simulink model "KEYPAD_FIN"  (R2019b)
settings: Solver=ode1  StartTime=0.0  StopTime=150  FixedStep=0.001  RelTol=1e-3  EnableMultiTasking=on
undefined symbols (not defined in the file or in its folder): sigbuilder_block
settings Model: ExtModeTrigDuration=2  Creator=estra  LastModifiedBy=fabia
settings DataIOCC: ReturnWorkspaceOutputs=off
settings OptimizationCC: MaxStackSize=64  EfficientTunableParamExpr=on
settings DebuggingCC: ParameterTunabilityLossMsg=error  FrameProcessingCompatibilityMsg=warning  NonCurrentReleaseOperatingPointMsg=warning  ArithmeticOperatorsInVariantConditions=warning
settings HardwareCC: ProdBitPerInt=16  ProdBitPerPointer=16  ProdBitPerSizeT=16  ProdBitPerPtrDiffT=16  ProdLargestAtomicFloat=None  ProdWordSize=8  ProdHWDeviceType=Atmel->AVR
settings SFSimCC: SimUseLocalCustomCode=off  MATLABDynamicMemAlloc=off  CustomCodeUndefinedFunction=UseInterfaceOnly
settings RTWCC: SystemTargetFile=ert.tlc  HardwareBoard=Arduino Uno  TLCOptions=-aInlineSetEventsForThisBaseRateFcn=TLC_FALSE -aSuppressMultiTaskScheduler=TLC_FALSE -aRateBasedStepFcn=1  TemplateMakefile=ert_default_tmf  GenerateReport=on  RTWUseLocalCustomCode=off  Toolchain=Arduino AVR  BuildConfiguration=Faster Runs  IncludeHyperlinkInReport=on  LaunchReport=on  GenerateTraceInfo=on  GenerateTraceReport=on  GenerateTraceReportSl=on  GenerateTraceReportSf=on  GenerateTraceReportEml=on
settings CodeAppCC: ForceParamTrailComments=on  IgnoreCustomStorageClasses=off  OperatorAnnotations=on  SimulinkDataObjDesc=on  SFDataObjDesc=on  MATLABFcnDesc=on  InsertBlockDesc=on  StateflowObjectComments=on  MATLABSourceComments=on
settings ERTTargetCC: MultiwordLength=2048  SupportContinuousTime=on  SupportVariableSizeSignals=on

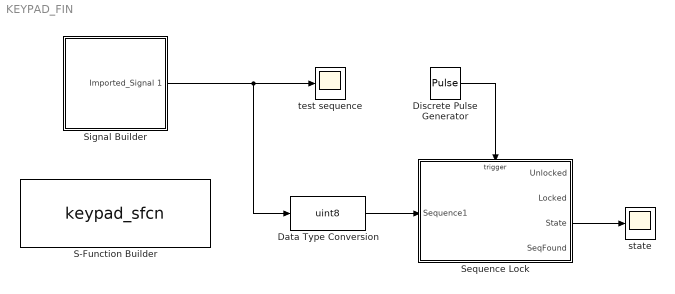
== system KEYPAD_FIN ==
  Data Type Conversion : DataTypeConversion  OutDataTypeStr=uint8
  Discrete Pulse Generator : DiscretePulseGenerator  PulseType=Time based  Period=0.01  PulseWidth=50
  S-Function Builder : S-Function  InitFcn=try, set_param(gcb,'FunctionName','keypad_sfcn'), end  FunctionName=keypad_sfcn  SFunctionModules=keypad_sfcn_wrapper  SFunctionDeploymentMode=off  EnableBusSupport=off  mask(S-Function Builder){}
      mask help: Simulink:masks:SFunctionBuilder_MD
      mask init:
      | val = [[.9  0.75 0.75 1 1 .9 .9 1]',[1 1 0.75 0.75 .9 .9 1 .9]'];try , sys = get_param(gcb,'SfunBuilderFcnName');if isempty(sys), sys = get_param(gcb,'FunctionName'); end,catch, sys = get_param(gcb,'FunctionName'); end
      settings: CopyFcn=set_param(gcbh,'LinkStatus','none')  PreSaveFcn=try, set_param(gcb,'FunctionName','keypad_sfcn'), end  OpenFcn=sfunctionwizard(gcbh)
      mask Display: plot(val(:,1),val(:,2)),disp(sys), port_label('output',1,'y0')
  Sequence Lock : Subsystem
  Signal Builder : Subsystem  Tag=STV Subsys  LoadFcn=sigbuilder_block('load');  StartFcn=sigbuilder_block('start');  StopFcn=sigbuilder_block('stop');  ClipboardFcn=sigbuilder_block('clipboard');  mask(Sigbuilder block){tuvar=[0:10]}
      mask help: Simulink:masks:SigbuilderBlock_MD
      mask init:
      | if ~strcmp(get_param(bdroot(gcbh),'SimulationStatus'),'stopped') tuvar = sigbuilder_block('maskInit'); end
      settings: CopyFcn=sigbuilder_block('copy');  DeleteFcn=sigbuilder_block('delete');  ModelCloseFcn=sigbuilder_block('modelClose');  PreSaveFcn=sigbuilder_block('preSave');  PauseFcn=sigbuilder_block('pause');  ContinueFcn=sigbuilder_block('continue');  NameChangeFcn=sigbuilder_block('namechange');  OpenFcn=sigbuilder_block('open',[6 114.75 1908 641.25 ]);  CloseFcn=sigbuilder_block('close');
      mask Display: plot(0, 0, 100, 100,[2, 2, 32, 32, 2], [68, 8, 8, 68, 68],[32, 2], [38, 38], [32, 19, 2],[53, 60, 44], [32, 17, 17, 2],[16, 16, 31, 31]);txt = getActiveGroup(gcbh);text(2, 100, txt,'verticalAlignment', 'top');
  state : Scope
  test sequence : Scope
  wires:
  Signal Builder/1(Imported_Signal 1) -> test sequence/1, Data Type Conversion/1
  Data Type Conversion/1 -> Sequence Lock/1(Sequence1)
  Discrete Pulse Generator/1 -> Sequence Lock/Trigger
  Sequence Lock/3(State) -> state/1

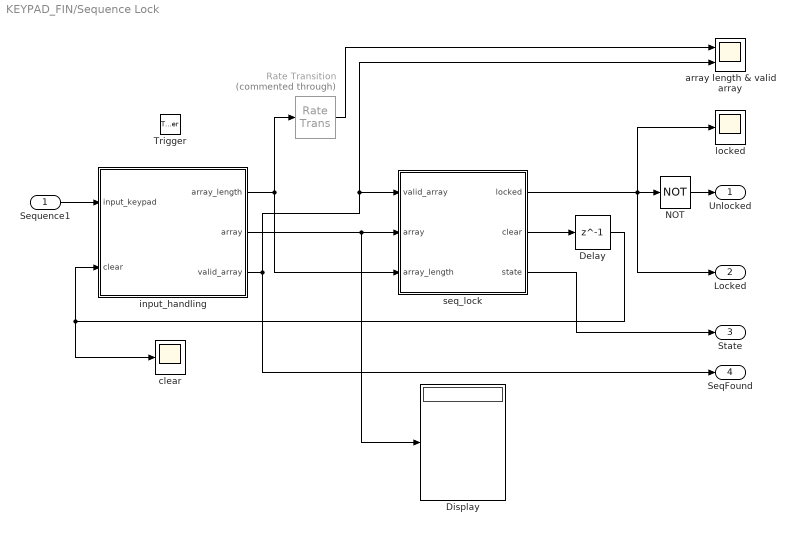
== system KEYPAD_FIN/Sequence Lock ==
  Sequence1 : Inport
  Trigger : TriggerPort  VariantControl=Variant  PortDimensions=1
  Delay : Delay  DelayLength=1  InitialCondition=0
  Display : Display
  NOT : Logic  Operator=NOT  IconShape=distinctive  AllPortsSameDT=off  OutDataTypeStr=boolean
  Rate Transition : RateTransition  Commented=through  OutPortSampleTimeOpt=Multiple of input port sample time  OutPortSampleTimeMultiple=50  OutPortSampleTime=1
  array length & valid array : Scope  NumInputPorts=2
  clear : Scope
  input_handling : Stateflow chart  TreatAsAtomicUnit=on
  locked : Scope
  seq_lock : Stateflow chart  TreatAsAtomicUnit=on
  Unlocked : Outport  VectorParamsAs1DForOutWhenUnconnected=off
  Locked : Outport  Port=2  VectorParamsAs1DForOutWhenUnconnected=off
  State : Outport  Port=3  VectorParamsAs1DForOutWhenUnconnected=off
  SeqFound : Outport  Port=4  VectorParamsAs1DForOutWhenUnconnected=off
  wires:
  input_handling/2(array) -> seq_lock/2(array), Display/1
  Rate Transition/1 -> array length & valid array/1
  seq_lock/1(locked) -> locked/1, Locked/1, NOT/1
  input_handling/1(array_length) -> seq_lock/3(array_length), Rate Transition/1
  input_handling/3(valid_array) -> SeqFound/1, seq_lock/1(valid_array), array length & valid array/2
  NOT/1 -> Unlocked/1
  seq_lock/3(state) -> State/1
  seq_lock/2(clear) -> Delay/1
  Delay/1 -> clear/1, input_handling/2(clear)
  Sequence1/1 -> input_handling/1(input_keypad)

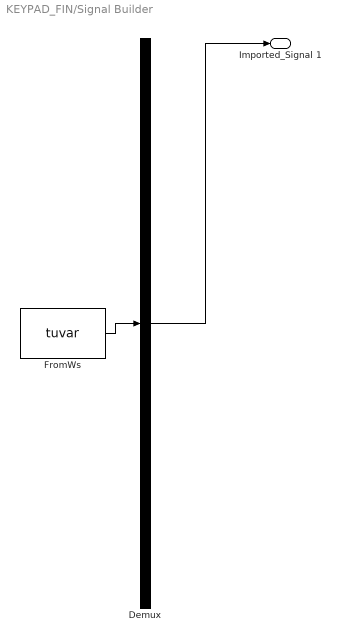
== system KEYPAD_FIN/Signal Builder ==
  Demux : Demux  Tag=STV Demux  Outputs=1
  FromWs : FromWorkspace  Tag=STV FromWs  VariableName=tuvar  SampleTime=0
      SigBuilderData=|
      | common.afterFinalStr = 'Extrapolate'
      | common.sampleTime = 0
      | dataSet.timeRange = [0 144]
      | dataSet.name = 'Imported_Group 1'
      | sbobj.Groups.Name = 'Imported_Group 1'
      | sbobj.Groups.Signals.Name = 'Imported_Signal 1'
      | sbobj.Groups.Signals.XData = [0 1 1 1.01 1.01 2 2 2.01 2.01 3 3 3.01 3.01 4 4 4.01 4.01 5 5 5.01 5.01 6 6 6.01 6.01 7 20 21 21 21.01 21.01 22 22 22.01 22.01 23 23 23.01 23.01 24 24 24.01 24.01 25 25 25.01 25.01 26 26 26.01 26.01 27 40 41 41 41.01 41.01 42 42 42.01 42.01 43 43 43.01 43.01 44 44 44.01 44.01 45 45 45.01 45.01 46 46 46.01 46.01 47 60 61 61 61.01 61.01 62 62 62.01 62.01 63 80 81 81 81.01 81.01 82 82 82.01 82.01 83 83 83.01 83.01 84 84 84.01 84.01 85 85 85.01 85.01 86 86 86.01 86.01 87 100 101 101 101.01 101.01 102 102 102.01 102.01 103 103 103.01 103.01 104 104 104.01 104.01 105 105 105.01 105.01 106 106 106.01 106.01 107 120 121 121 121.01 121.01 122 122 122.01 122.01 123 123 123.01 123.01 124 140 141 141 141.01 141.01 142 142 142.01 142.01 143 143 143.01 143.01 144]
      | sbobj.Groups.Signals.YData = [0 0 49 49 0 0 48 48 0 0 48 48 0 0 49 49 0 0 50 50 0 0 42 42 0 0 0 0 50 50 0 0 48 48 0 0 53 53 0 0 54 54 0 0 50 50 0 0 35 35 0 0 0 0 49 49 0 0 48 48 0 0 48 48 0 0 49 49 0 0 50 50 0 0 35 35 0 0 0 0 42 42 0 0 42 42 0 0 0 0 50 50 0 0 48 48 0 0 53 53 0 0 54 54 0 0 50 50 0 0 35 35 0 0 0 0 49 49 0 0 48 48 0 0 48 48 0 0 49 49 0 0 50 50 0 0 35 35 0 0 0 0 49 49 0 0 48 48 0 0 42 42 0 0 0 0 49 49 0 0 48 48 0 0 35 35 0 0]
      | sbobj.Groups.TimeRange = [0 107]
  Imported_Signal 1 : Outport  Tag=STV Outport
  wires:
  Demux/1 -> Imported_Signal 1/1
  FromWs/1 -> Demux/1

== stateflow chart KEYPAD_FIN/Sequence Lock/input_handling ==
  settings: updateMethod=DISCRETE
  state INIT
    array_length = 0;
    array = uint8([]);
    valid_array = false;
  state CONCATENATE
    entry:
    array = cat(1, array, input_keypad);
    array_length = uint8(length(array));
    during:
    exit:
  state IDLE
    %Do absolutely nothing :D
  state STRING_FINSHED
    entry:
    valid_array = true;
    array_length = uint8(length(array));
    during:
    exit:
  (default) -> INIT
  IDLE -> INIT [order 2] : [after(7,sec) || clear==true]
  STRING_FINSHED -> INIT [order 2] : [clear == true]
  CONCATENATE -> INIT [order 1] : [array_length > 8 || clear == true]
  INIT -> IDLE [order 1] : [input_keypad == 0]
  INIT -> CONCATENATE [order 2]
  IDLE -> CONCATENATE [order 1] : [(input_keypad <= '9' && input_keypad >= '0') || input_keypad == '*'|| input_keypad == '#']
  CONCATENATE -> (junction 32) [order 3] : [hasChangedTo(input_keypad,uint8(0))]
  CONCATENATE -> STRING_FINSHED [order 2] : [(array(array_length)=='*' || array(array_length)=='#') && array_length >= 2]
  (junction 32) -> IDLE
  STRING_FINSHED -> (junction 32) [order 1] : [hasChangedTo(input_keypad,uint8(0))]
  data: input_keypad input uint8 size=1 [0..254]; array_length output uint8 size=1; array output uint8 size=9; clear input boolean size=1; valid_array output boolean size=1

== stateflow chart KEYPAD_FIN/Sequence Lock/seq_lock ==
  state INIT
    locked = false;
    clear = false;
    password = [];
    password_old = [];
    keep_password = false;
    state = 0;
  state IDLE
    clear = false;
    locked = false;
    state = 1;
  state LOCKED
    entry:
    if(keep_password)
    password = password_old;
    else
    password = array;
    end
    password_length = uint8(length(password));
    clear = true;
    during:
    clear = false;
    locked = true;
    state = 2;
    exit:
    password_old = password;
  state WRONG_PASS
    %led_red blinken
    state = 5;
    clear = true;
    keep_password = true;
  state UNLOCKED
    entry:
    clear = true;
    during:
    clear = false;
    locked = false;
    keep_password = false;
    state = 4;
  (default) -> INIT
  INIT -> IDLE
  IDLE -> LOCKED : [valid_array && (array(array_length) == '*') && (~(array(array_length - 1) == '*'))]{clear = true, password = array}
  (junction 86) -> LOCKED [order 2] : {keep_password = false}
  (junction 86) -> LOCKED [order 1] : [(array(array_length) == '*') && (array(array_length - 1) == '*') && array_length == 2]{keep_password = true}
  UNLOCKED -> (junction 86) : [valid_array]
  (junction 78) -> LOCKED [order 3]
  WRONG_PASS -> LOCKED : [after(3,sec)]
  LOCKED -> (junction 78) : [valid_array && (array(array_length) == '#')]
  (junction 78) -> WRONG_PASS [order 2] : [compare(array, array_length, password, password_length) == 0]
  (junction 78) -> UNLOCKED [order 1] : [compare(array, array_length, password, password_length) == 1]
  data: password local uint8 size=9; locked output boolean size=1; valid_array input boolean size=1; array input uint8 size=9; array_length input uint8 size=1; clear output boolean size=1; password_length local uint8 size=1; password_old local uint8 size=9; keep_password local boolean size=1; state output uint8 size=1
